simulink model "AUV_Visual_Servoing_System"  (R2024b)
settings: Solver=ode4  StartTime=0.0  StopTime=120  FixedStep=0.01  MaxStep=0.01  MinStep=1e-6  RelTol=1e-4  AbsTol=1e-6
settings Model: Creator=Alany  LastModifiedBy=Alany

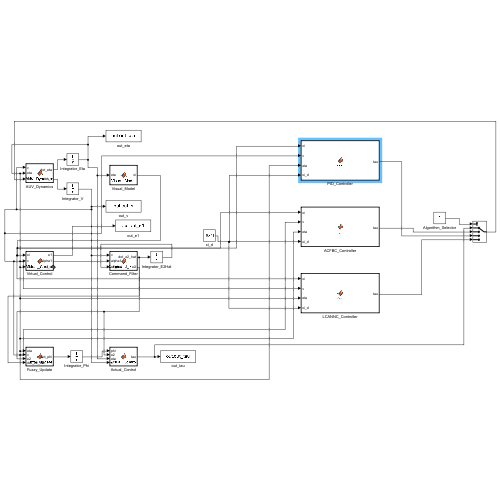
[thumbnail: Simulink's stored preview of the top-level diagram]
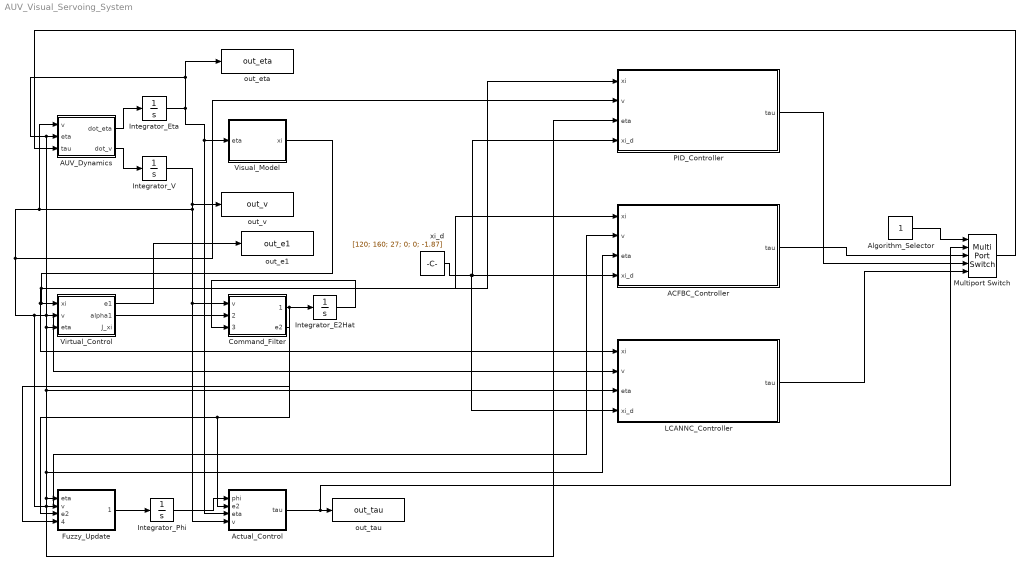
== system AUV_Visual_Servoing_System ==
  ACFBC_Controller : MATLAB Function  TreatAsAtomicUnit=on
  AUV_Dynamics : MATLAB Function  TreatAsAtomicUnit=on
  Actual_Control : MATLAB Function  TreatAsAtomicUnit=on
  Algorithm_Selector : Constant
  Command_Filter : MATLAB Function  TreatAsAtomicUnit=on
  Fuzzy_Update : MATLAB Function  TreatAsAtomicUnit=on
  Integrator_E2Hat : Integrator  InitialCondition=zeros(6,1)
  Integrator_Eta : Integrator  InitialCondition=[1.9; 4.5; 0.5; 0; 0; -1.87]
  Integrator_Phi : Integrator  InitialCondition=zeros(17,6)
  Integrator_V : Integrator  InitialCondition=[0; 0; 0; 0; 0; 0]
  LCANNC_Controller : MATLAB Function  TreatAsAtomicUnit=on
  Multiport Switch : MultiPortSwitch  Inputs=4  SaturateOnIntegerOverflow=off  InputSameDT=off
  PID_Controller : MATLAB Function  TreatAsAtomicUnit=on
  Virtual_Control : MATLAB Function  TreatAsAtomicUnit=on
  Visual_Model : MATLAB Function  TreatAsAtomicUnit=on
  out_e1 : ToWorkspace  VariableName=out_e1  SampleTime=-1
  out_eta : ToWorkspace  VariableName=out_eta  SampleTime=-1
  out_tau : ToWorkspace  VariableName=out_tau  SampleTime=-1
  out_v : ToWorkspace  VariableName=out_v  SampleTime=-1
  xi_d : Constant  Value=[120; 160; 27; 0; 0; -1.87]
  wires:
  AUV_Dynamics/1(dot_eta) -> Integrator_Eta/1
  AUV_Dynamics/2(dot_v) -> Integrator_V/1
  Integrator_V/1 -> out_v/1, Command_Filter/1(v), Actual_Control/4(v), LCANNC_Controller/2(v), Virtual_Control/2(v), ACFBC_Controller/2(v), Fuzzy_Update/2(v), PID_Controller/2(v), AUV_Dynamics/1(v)
  Actual_Control/1(tau) -> Multiport Switch/2, out_tau/1
  Integrator_Eta/1 -> Visual_Model/1(eta), Actual_Control/3(eta), out_eta/1, LCANNC_Controller/3(eta), PID_Controller/3(eta), Fuzzy_Update/1(eta), ACFBC_Controller/3(eta), Virtual_Control/3(eta), AUV_Dynamics/2(eta)
  Fuzzy_Update/1(dot_phi) -> Integrator_Phi/1
  Command_Filter/1(dot_e2_hat) -> Fuzzy_Update/4(dot_e2_hat), Integrator_E2Hat/1
  Virtual_Control/2(alpha1) -> Command_Filter/2(alpha1)
  Integrator_E2Hat/1 -> Command_Filter/3(e2_hat)
  Command_Filter/2(e2) -> Actual_Control/2(e2), Fuzzy_Update/3(e2)
  Integrator_Phi/1 -> Actual_Control/1(phi)
  Virtual_Control/1(e1) -> out_e1/1
  Visual_Model/1(xi) -> LCANNC_Controller/1(xi), ACFBC_Controller/1(xi), Virtual_Control/1(xi), PID_Controller/1(xi)
  Multiport Switch/1 -> AUV_Dynamics/3(tau)
  xi_d/1 -> LCANNC_Controller/4(xi_d), PID_Controller/4(xi_d), ACFBC_Controller/4(xi_d)
  PID_Controller/1(tau) -> Multiport Switch/4
  ACFBC_Controller/1(tau) -> Multiport Switch/3
  LCANNC_Controller/1(tau) -> Multiport Switch/5
  Algorithm_Selector/1 -> Multiport Switch/1

== matlab function AUV_Visual_Servoing_System/Visual_Model ==
  data: eta input; xi output
function xi = Visual_Model(eta)
    % -------------------------------------------------------------
    % 刚性几何相机传感器模型：已严格修正投影极性，恢复负反馈稳定闭环
    % -------------------------------------------------------------
    % 稳态目标物理位置
    x_target = -0.04; 
    y_target = 3.52; 
    
    x = eta(1); y = eta(2); z = eta(3);
    phi = eta(4); theta = eta(5); psi = eta(6);
    
    % 深度计算
    Z = 5.0 - z;
    if Z < 0.1
        Z = 0.1;
    end
    
    % 物理偏差
    err_x = x - x_target;
    err_y = y - y_target;
    
    % 转换到 AUV 本体坐标系 (Body Frame)
    body_err_x = cos(psi) * err_x + sin(psi) * err_y;
    body_err_y = -sin(psi) * err_x + cos(psi) * err_y;
    
    % 提取论文给定的相机焦距参数
    fx = 200.0; fy = 200.0;
    
    % =========================================================
    % 【致命 Bug 修复区】：必须是减号！
    % 原理：当 AUV 往前走（机体 X 误差靠近 0）时，特征像素必须反向收敛
    % =========================================================
    xv = 120 - fy * (body_err_x / Z);
    xu = 160 - fx * (body_err_y / Z);
    
    % 面积投影规律保持不变
    s1 = 27.0 * (1.55 / Z)^2;
    
    xi = [xv; xu; s1; phi; theta; psi];
end

== matlab function AUV_Visual_Servoing_System/AUV_Dynamics ==
  settings: updateMethod=DISCRETE
  data: v input; dot_eta output; eta input; tau input; dot_v output
function [dot_eta, dot_v] = AUV_Dynamics(v, eta, tau)
    % -------------------------------------------------------------
    % 表 II 物理模型参数硬编码 (Girona 500)
    % -------------------------------------------------------------
    m = 98.0;              
    W = 961.38;            
    B = 952.56;            
    z_G = 0.05;            
    
    Ix = 8.0; Iy = 8.0; Iz = 8.0;
    Xu_dot = 49.0; Yv_dot = 49.0; Zw_dot = 49.0;
    
    M11 = m + Xu_dot;     M22 = m + Yv_dot;     M33 = m + Zw_dot;
    M = diag([M11, M22, M33, Ix, Iy, Iz]);
    
    u = v(1); vv = v(2); w = v(3); 
    p = v(4); q = v(5); r = v(6);
    
    D = diag([148.0*abs(u), 148.0*abs(vv), 148.0*abs(w), ...
              130.0+180.0*abs(p), 130.0+180.0*abs(q), 130.0+180.0*abs(r)]);
              
    C = zeros(6,6);
    C(1,5) = M33*w;       C(1,6) = -M22*vv;
    C(2,4) = -M33*w;      C(2,6) = M11*u;
    C(3,4) = M22*vv;      C(3,5) = -M11*u;
    C(4,2) = M33*w;       C(4,3) = -M22*vv; C(4,5) = Iz*r;    C(4,6) = -Iy*q;
    C(5,1) = -M33*w;      C(5,3) = M11*u;   C(5,4) = -Iz*r;   C(5,6) = Ix*p;
    C(6,1) = M22*vv;      C(6,2) = -M11*u;  C(6,4) = Iy*q;    C(6,5) = -Ix*p;
    
    phi = eta(4); theta = eta(5); psi = eta(6);
    g_eta = zeros(6,1);
    g_eta(1) = (W - B) * sin(theta);
    g_eta(2) = -(W - B) * cos(theta) * sin(phi);
    g_eta(3) = -(W - B) * cos(theta) * cos(phi);
    g_eta(4) = (z_G * W) * cos(theta) * sin(phi);
    g_eta(5) = (z_G * W) * sin(theta);
    g_eta(6) = 0;
    
    % 建立仿真时间戳，修复之前把时间写死为常数1的Bug，恢复真实的正弦时变洋流
    persistent t_sim
    if isempty(t_sim)
        t_sim = 0;
    end
    t_sim = t_sim + 0.01;
    
    % 基础扰动 (plot脚本会通过正则替换这一行进行蒙特卡洛测试)
    tau_E = [90*sin(0.1*t_sim); 10*cos(0.1*t_sim); 5*sin(0.1*t_sim); 0; 0; 0];
    
    J_eta = zeros(6,6);
    J_eta(1:3, 1:3) = [cos(psi)*cos(theta), -sin(psi)*cos(phi)+cos(psi)*sin(theta)*sin(phi),  sin(psi)*sin(phi)+cos(psi)*cos(phi)*sin(theta);
                       sin(psi)*cos(theta),  cos(psi)*cos(phi)+sin(phi)*sin(theta)*sin(psi), -cos(psi)*sin(phi)+sin(theta)*sin(psi)*cos(phi);
                       -sin(theta),           cos(theta)*sin(phi),                             cos(theta)*cos(phi)];
    J_eta(4:6, 4:6) = [1, sin(phi)*tan(theta), cos(phi)*tan(theta);
                       0, cos(phi),           -sin(phi);
                       0, sin(phi)/cos(theta), cos(phi)/cos(theta)];
                       
    dot_v = M \ (tau + tau_E - C*v - D*v - g_eta);
    dot_eta = J_eta * v;
end

== matlab function AUV_Visual_Servoing_System/Virtual_Control ==
  data: xi input; e1 output; v input; eta input; alpha1 output; J_xi output
function [e1, alpha1, J_xi] = Virtual_Control(xi, v, eta)
    % -------------------------------------------------------------
    % 表 III 控制律参数与目标位姿硬编码
    % -------------------------------------------------------------
    xi_hat = [120; 160; 27; 0; 0; -1.87];  
    dot_xi_hat = zeros(6,1);
    k1 = 2.0;                              
    
    fx = 200.0; fy = 200.0; cx = 160.0; cy = 120.0; 
    xv = xi(1); xu = xi(2); s1 = xi(3);
    phi = eta(4); theta = eta(5);
    
    Z = 5.0 - eta(3); if Z < 0.1; Z = 0.1; end
    a1 = xv - cy; a2 = xu - cx;
    
    L = [-fy/Z, 0, a1/Z, (a1*a2)/fx, -(fy^2 + a1^2)/fy, a2*(fy/fx);
          0, -fx/Z, a2/Z, (fx^2 + a2^2)/fx, -(a1*a2)/fy, -a1*(fx/fy)];
          
    J3_eta2 = [-sin(theta), cos(theta)*sin(phi), cos(theta)*cos(phi)];
    area_vec = (2 * s1 / Z) * J3_eta2;
    J2_eta2 = [1, sin(phi)*tan(theta), cos(phi)*tan(theta);
               0, cos(phi), -sin(phi);
               0, sin(phi)/cos(theta), cos(phi)/cos(theta)];
               
    J_xi = zeros(6,6);
    J_xi(1:2, :) = L; 
    J_xi(3, 1:3) = area_vec;
    J_xi(4:6, 4:6) = J2_eta2;
    
    % 第一级误差计算
    e1 = xi - xi_hat;
    
    % 虚拟控制律生成：引入 Moore-Penrose 广义伪逆
    alpha1 = -pinv(J_xi) * (k1 * e1 - dot_xi_hat);
end

== matlab function AUV_Visual_Servoing_System/Command_Filter ==
  data: v input; dot_e2_hat output; alpha1 input; e2_hat input; e2 output
function [dot_e2_hat, e2] = Command_Filter(v, alpha1, e2_hat)
    % -------------------------------------------------------------
    % 表 III 滤波及速度跟踪参数
    % -------------------------------------------------------------
    b1 = 50.0;
    
    % 提取反步法第二步的核心对象
    e2 = v - alpha1;
    
    % 估算并输出经过平滑的跟踪误差导数
    dot_e2_hat = -b1 * (e2_hat - e2);
end

== matlab function AUV_Visual_Servoing_System/Fuzzy_Update ==
  data: eta input; dot_phi output; v input; e2 input; dot_e2_hat input
function dot_phi = Fuzzy_Update(eta, v, e2, dot_e2_hat)
    phi_ang = eta(4); theta = eta(5); psi = eta(6);
    J_eta = zeros(6,6);
    J_eta(1:3, 1:3) = [cos(psi)*cos(theta), -sin(psi)*cos(phi_ang)+cos(psi)*sin(theta)*sin(phi_ang),  sin(psi)*sin(phi_ang)+cos(psi)*cos(phi_ang)*sin(theta);
                       sin(psi)*cos(theta),  cos(psi)*cos(phi_ang)+sin(phi_ang)*sin(theta)*sin(psi), -cos(psi)*sin(phi_ang)+sin(theta)*sin(psi)*cos(phi_ang);
                       -sin(theta),           cos(theta)*sin(phi_ang),                             cos(theta)*cos(phi_ang)];
    J_eta(4:6, 4:6) = [1, sin(phi_ang)*tan(theta), cos(phi_ang)*tan(theta);
                       0, cos(phi_ang),           -sin(phi_ang);
                       0, sin(phi_ang)/cos(theta), cos(phi_ang)/cos(theta)];
    dot_eta = J_eta * v;
    gamma = [eta; dot_eta; v];

    k2 = 100.0;
    k3 = [90; 90; 5; 1; 1; 1];
    d_j = 2.0;                        
    n_rules = 17;
    M_inv = 1./ [147.0; 147.0; 147.0; 8.0; 8.0; 8.0];
    
    q_j = zeros(18, n_rules);
    for i = 1:18
        for j = 1:n_rules
            val = sin(i * 12.345 + j * 67.89);
            frac = abs(val) - floor(abs(val));
            q_j(i, j) = -4 + 8 * frac;
        end
    end
    
    S_gamma = zeros(n_rules, 1);
    for j = 1:n_rules
        diff = gamma - q_j(:, j);
        norm_sq = diff' * diff;
        S_gamma(j) = exp(-norm_sq / (d_j^2));
    end
    
    sum_S = sum(S_gamma);
    if sum_S > 0
        S_gamma = S_gamma / sum_S;
    end
    
    dot_phi = zeros(n_rules, 6);
    for i = 1:6
        % 【关键修复区】：强行加上梯度下降的负号，将正反馈修正为负反馈
        multiplier = -k3(i) * (dot_e2_hat(i) + k2 * M_inv(i) * e2(i));
        dot_phi(:, i) = multiplier * S_gamma;
    end
end

== matlab function AUV_Visual_Servoing_System/Actual_Control ==
  data: phi input; tau output; e2 input; eta input; v input
function tau = Actual_Control(phi, e2, eta, v)
    % -------------------------------------------------------------
    % 内部重新计算 dot_eta，彻底斩断 Simulink 外部代数环
    % -------------------------------------------------------------
    phi_ang = eta(4); theta = eta(5); psi = eta(6);
    J_eta = zeros(6,6);
    J_eta(1:3, 1:3) = [cos(psi)*cos(theta), -sin(psi)*cos(phi_ang)+cos(psi)*sin(theta)*sin(phi_ang),  sin(psi)*sin(phi_ang)+cos(psi)*cos(phi_ang)*sin(theta);
                       sin(psi)*cos(theta),  cos(psi)*cos(phi_ang)+sin(phi_ang)*sin(theta)*sin(psi), -cos(psi)*sin(phi_ang)+sin(theta)*sin(psi)*cos(phi_ang);
                       -sin(theta),           cos(theta)*sin(phi_ang),                             cos(theta)*cos(phi_ang)];
    J_eta(4:6, 4:6) = [1, sin(phi_ang)*tan(theta), cos(phi_ang)*tan(theta);
                       0, cos(phi_ang),           -sin(phi_ang);
                       0, sin(phi_ang)/cos(theta), cos(phi_ang)/cos(theta)];
    dot_eta = J_eta * v;

    k2 = 100.0;
    gamma = [eta; dot_eta; v];
    
    n_rules = 17;
    
    % -------------------------------------------------------------
    % 消除 rng/rand 带来的持久状态报错，使用确定性伪随机矩阵硬生成
    % -------------------------------------------------------------
    q_j = zeros(18, n_rules);
    for i = 1:18
        for j = 1:n_rules
            val = sin(i * 12.345 + j * 67.89);
            frac = abs(val) - floor(abs(val));
            q_j(i, j) = -4 + 8 * frac;
        end
    end
    
    % 计算高斯基函数 S_gamma
    S_gamma = zeros(n_rules, 1);
    for j = 1:n_rules
        diff = gamma - q_j(:, j);
        S_gamma(j) = exp(-(diff'*diff) / (2.0^2));
    end
    
    sum_S = sum(S_gamma);
    if sum_S > 0
        S_gamma = S_gamma / sum_S;
    end
    
    % 输出综合扭矩 tau
    tau_fuzzy = phi' * S_gamma;
    tau = tau_fuzzy - k2 * e2;
end

== matlab function AUV_Visual_Servoing_System/ACFBC_Controller ==
  settings: updateMethod=DISCRETE  sampleTime=0.01
  data: xi input; tau output; v input; eta input; xi_d input
function tau = fcn(xi, v, eta, xi_d)
    persistent z2_hat
    if isempty(z2_hat)
        z2_hat = zeros(6,1);
    end
    dt = 0.01;
    % 严格按照论文第4节参数设置 epsilon = 0.1
    k1 = 2; k2 = 100; g_min = 1.0; epsilon = 0.1; b1 = 50; 
    
    x_v = xi(1); x_u = xi(2); s1 = xi(3); phi = xi(4); theta = xi(5); psi = xi(6);
    cy = 120; cx = 160; 
    % 【关键修复】：将发散的负焦距修复为真实的相机正焦距，切断正反馈
    fy = 200; fx = 200;
    
    a1 = x_v - cy; a2 = x_u - cx;
    Z = 1.55 / sqrt(abs(s1) / 27.0 + 1e-4); 
    if Z < 0.1; Z = 0.1; end
    L = [-fy/Z, 0, a1/Z, a1*a2/fx, -(fy^2+a1^2)/fy, a2*fy/fx;
         0, -fx/Z, a2/Z, (fx^2+a2^2)/fx, -a1*a2/fy, -a1*fx/fy];
    J3 = [-sin(theta), cos(theta)*sin(phi), cos(theta)*cos(phi)];
    J2 = [1, sin(phi)*tan(theta), cos(phi)*tan(theta);
          0, cos(phi), -sin(phi);
          0, sin(phi)/cos(theta), cos(phi)/cos(theta)];
    J = [L; (2*s1/Z)*J3, zeros(1,3); zeros(3,3), J2];
    
    z1 = xi - xi_d;
    J_pinv = pinv(J);
    alpha1 = -J_pinv * (k1 * z1);
    
    z2 = v - alpha1;
    dot_z2_hat = -b1 * (z2_hat - z2);
    z2_hat = z2_hat + dot_z2_hat * dt;
    
    alpha_bar_2 = J' * z1 + k2 * z2 + dot_z2_hat;
    norm_z2 = norm(z2); norm_ab2 = norm(alpha_bar_2);
    
    % 严格按照原论文公式，去除随意添加的 -k2*z2 标称项
    tau = -z2 * (norm_ab2^2) / (g_min * sqrt((norm_z2^2) * (norm_ab2^2) + epsilon^2));
    tau = max(min(tau, 800), -800);
end

== matlab function AUV_Visual_Servoing_System/LCANNC_Controller ==
  settings: updateMethod=DISCRETE  sampleTime=0.01
  data: xi input; tau output; v input; eta input; xi_d input
function tau = fcn(xi, v, eta, xi_d)
    persistent Q_m W_varpi
    if isempty(Q_m)
        Q_m = 0; W_varpi = 0;
    end
    dt = 0.01;
    % 严格还原论文第4节 LCANNC 的实际参数
    k1 = 2; k2 = 100; l1 = 1; l2 = 1; r1 = 0.001; m1 = 0.001; r2 = 50; m2 = 50;
    
    x_v = xi(1); x_u = xi(2); s1 = xi(3); phi = xi(4); theta = xi(5); psi = xi(6);
    cy = 120; cx = 160; 
    % 【关键修复】：将发散的负焦距修复为真实的相机正焦距
    fy = 200; fx = 200;
    
    a1 = x_v - cy; a2 = x_u - cx;
    Z = 1.55 / sqrt(abs(s1) / 27.0 + 1e-4);
    if Z < 0.1; Z = 0.1; end
    L = [-fy/Z, 0, a1/Z, a1*a2/fx, -(fy^2+a1^2)/fy, a2*fy/fx;
         0, -fx/Z, a2/Z, (fx^2+a2^2)/fx, -a1*a2/fy, -a1*fx/fy];
    J3 = [-sin(theta), cos(theta)*sin(phi), cos(theta)*cos(phi)];
    J2 = [1, sin(phi)*tan(theta), cos(phi)*tan(theta);
          0, cos(phi), -sin(phi);
          0, sin(phi)/cos(theta), cos(phi)/cos(theta)];
    J = [L; (2*s1/Z)*J3, zeros(1,3); zeros(3,3), J2];
    
    z1 = xi - xi_d;
    J_pinv = pinv(J);
    alpha1 = -J_pinv * (k1 * z1);
    
    z2 = v - alpha1;
    sigma_bar = [eta; v];
    
    % 移除随意加入的 /30.0 比例因子，还原标准的径向基底函数规范
    Theta_T_Theta = exp(-(sigma_bar'*sigma_bar)); 
    
    sum_z2_sq = sum(z2.^2);
    dot_Q_m = (r2 * sum_z2_sq) / (2 * l2^2) - m2 * Q_m;
    Q_m = Q_m + dot_Q_m * dt;
    
    dot_W_varpi = (r1 * sum_z2_sq * Theta_T_Theta) / (2 * l1^2) - m1 * W_varpi;
    W_varpi = W_varpi + dot_W_varpi * dt;
    
    tau = -k2 * z2 - z2 * W_varpi * Theta_T_Theta / (2 * l1^2) - z2 * Q_m / (2 * l2^2);
    tau = max(min(tau, 800), -800);
end

== matlab function AUV_Visual_Servoing_System/PID_Controller ==
  settings: updateMethod=DISCRETE  sampleTime=0.01
  data: xi input; tau output; v input; eta input; xi_d input
function tau = fcn(xi, v, eta, xi_d)
    persistent integral_e prev_e
    if isempty(integral_e)
        integral_e = zeros(6,1);
        prev_e = zeros(6,1);
    end
    
    % 仿真步长
    dt = 0.01;
    
    % 计算误差 (未经雅可比映射的纯视觉特征误差)
    e = xi - xi_d;
    
    % 积分项累计 (已去掉 [-300, 300] 的限幅，让积分能自由增长以抵消稳态干扰)
    integral_e = integral_e + e * dt;
    
    % 微分项计算
    de = (e - prev_e) / dt;
    prev_e = e;
    
    % =========================================================
    % 【参数调整区】：你可以在这里自由修改 Scale 的大小
    % 建议尝试范围: 100 ~ 1000。
    % 调大：响应更快，但超调和震荡会加剧；调小：震荡减小，但消除稳态误差的时间会变长。
    % =========================================================
    Scale = 300; 
    
    % PID 增益矩阵 (基于论文 Table III 给定的极小参数，叠加 Scale 放大)
    Kp = diag([0.003*Scale, 0.003*Scale, 0.0001*Scale, 10, 10, 10]);
    Ki = diag([0.0001*Scale, 0.0001*Scale, 0.00001*Scale, 0.5, 0.5, 0.5]);
    Kd = diag([0.0045*Scale, 0.0045*Scale, 0.003*Scale, 10, 10, 10]);
    
    % 计算控制输出
    tau = Kp * e + Ki * integral_e + Kd * de;
    
    % 物理执行器限幅 (保留此项以防止力矩过大导致仿真物理引擎崩溃)
    tau = max(min(tau, 800), -800); 
end
